simulink model "Cv_05_Problem_1"  (R2022b)
settings: Solver=VariableStepAuto  StartTime=0.0  StopTime=200  MaxStep=0.01  MinStep=0.001  RelTol=1e-3
libraries: slpidlib x5
settings Model: Creator=honza  LastModifiedBy=honza

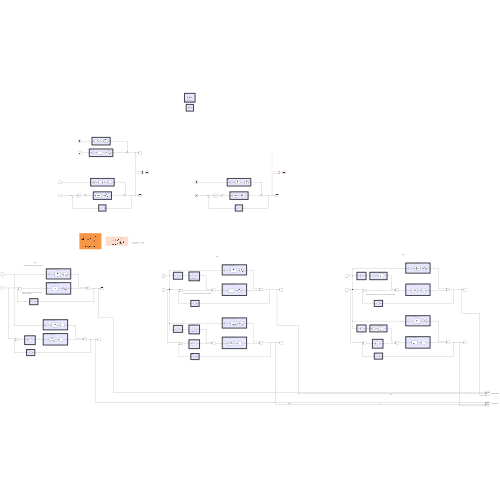
[thumbnail: Simulink's stored preview of the top-level diagram]
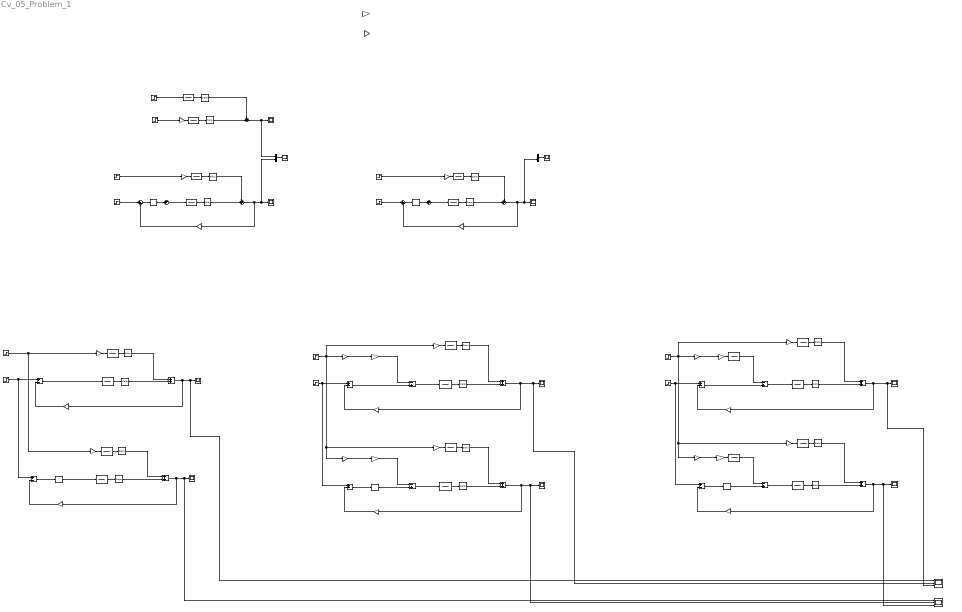
== system Cv_05_Problem_1 ==
  note: REGULOVANÁ
  note: NEREGULOVANÁ
  note: r0 = 0.35*15/(0.6*2)	= 4.375
      | Ti = 1.2*15			= 18
  note: Gt
  note: Gs
  note: Gd
  note: Gz
  note: Gs
  note: Gd
  note: Gf = -1/3
      |
      |
      |
      |
      | Gf = Gd/(Gt * Gs)
      | Ale jen to zesílení K
  note: Gs
  note: Gd
  note: Gz
  note: Gz = 1
  note: Gd = -(0.2 * e^-2s)/(10s + 1)
  note: Gt = 1
  note: Gz = 1
  note: Bod 2
  note: Bod 0
  note: Regulator vynechám, abych si ho mohl dopočítat a věděl co do něj zadat
  note: Bod 1
  note: Gd = -(0.2 * e^-2s)/(10s + 1)
  note: Gs = (0.6 * e^-2s)/(15s + 1)
  note: Gd = -(0.2 * e^-2s)/(10s + 1)
  note: Gr
  note: Gz = 1
  note: Gr
  note: Gt = 1
  note: Gf = -1/3
      |
      |
      |
      |
      | Gf = Gd/(Gt * Gs)
      | Ale jen to zesílení K
  note: Gz = 1
  note: Gz = 1
  note: Gs = (0.6 * e^-2s)/(15s + 1)
  note: Gs = (0.6 * e^-2s)/(15s + 1)
  note: Gd = -(0.2 * e^-2s)/(10s + 1)
  note: Gf = -1/3
      |
      |
      |
      |
      | Gf = Gd/(Gt * Gs)
      | Ale jen to zesílení K
  note: Gs = (0.6 * e^-2s)/(15s + 1)
  note: Regulator vynechám, abych si ho mohl dopočítat a věděl co do něj zadat
  note: Gs = (0.6 * e^-2s)/(15s + 1)
  note: Gz = 1
  note: Gd = -(0.2 * e^-2s)/(10s + 1)
  note: Gf = -1/3((15s + 1)/(10s + 1))
      |
      |
      |
      |
      | Gf = Gd/(Gt * Gs)
  note: Gf = -1/3((15s + 1)/(10s + 1))
  note: Gr
  note: Gd = -(0.2 * e^-2s)/(10s + 1)
  note: Gs = (0.6 * e^-2s)/(15s + 1)
  note: Gt = 1
  note: Gt = 1
  note: Otestujeme funkcnost bez kompenzace Gf (Gf = 0)
  note: Regulator vynechám, abych si ho mohl dopočítat a věděl co do něj zadat
  Add{,3,7,13} (4 alike) : Sum  Inputs=-+
  Add{1,4,6,9,11,14} (6 alike) : Sum
  Add{2,5,8,10,12,15} (6 alike) : Sum  Inputs=+-
  D3 : Step  Time=100  SampleTime=0
  D4 : Step  Time=100  SampleTime=0
  D5 : Step  Time=100  SampleTime=0
  Gain{,1,4,7..8,10,13,15..16,20..21,24,26} (13 alike) : Gain
  Gain{5,11,18..19,22} (5 alike) : Gain  Gain=-1/3
  Gain{2..3,6,9,12,14,17,23,25} (9 alike) : Gain  Gain=-1
  Mux : Mux  Inputs=2
  Mux1 : Mux  Inputs=2
  PID Controller{,1..4} (5 alike) : slpidlib/PID Controller  Controller=PI  Form=Ideal  TimeDomain=Continuous-time  UseExternalTs=off  SampleTime=-1  IntegratorMethod=Forward Euler  FilterMethod=Forward Euler  ControllerParametersSource=internal  P=4.375  I=1/18  UseKiTs=off  D=0  N=100  UseFilter=on  TunerSelectOption=Transfer Function Based (PID Tuner App)  InitialConditionSource=internal  InitialConditionForIntegrator=0  InitialConditionForFilter=0  DifferentiatorICPrevScaledInput=0  ExternalReset=none  TrackingMode=off  Kt=1  LimitOutput=off  SatLimitsSource=internal  UpperSaturationLimit=inf  LowerSaturationLimit=-inf  LinearizeAsGain=on  AntiWindupMode=none  Kb=1  LimitIntegrator=off  UpperIntegratorSaturationLimit=inf  LowerIntegratorSaturationLimit=-inf  POutMin=[]  POutMax=[]  IOutMin=[]  IOutMax=[]  DOutMin=[]  DOutMax=[]  NOutMin=[]  NOutMax=[]  SumOutMin=[]  SumOutMax=[]  SaturationOutMin=[]  SaturationOutMax=[]  PParamMin=[]  PParamMax=[]  IParamMin=[]  IParamMax=[]  DParamMin=[]  DParamMax=[]  NParamMin=[]  NParamMax=[]  KbParamMin=[]  KbParamMax=[]  KtParamMin=[]  KtParamMax=[]  KbOutMin=[]  KbOutMax=[]  KtOutMin=[]  KtOutMax=[]  IntegratorOutMin=[]  IntegratorOutMax=[]  FilterOutMin=[]  FilterOutMax=[]  SumI1OutMin=[]  SumI1OutMax=[]  SumI2OutMin=[]  SumI2OutMax=[]  SumI3OutMin=[]  SumI3OutMax=[]  SumI4OutMin=[]  SumI4OutMax=[]  SumDOutMin=[]  SumDOutMax=[]  DifferentiatorOutMin=[]  DifferentiatorOutMax=[]  FilterDiffOutCoefMin=[]  FilterDiffOutCoefMax=[]  ReciprocalOutMin=[]  ReciprocalOutMax=[]  SumDenOutMin=[]  SumDenOutMax=[]  SumNumOutMin=[]  SumNumOutMax=[]  DivideOutMin=[]  DivideOutMax=[]  UdiffTsProdOutMin=[]  UdiffTsProdOutMax=[]  NTsProdOutMin=[]  NTsProdOutMax=[]  UintegralTsProdOutMin=[]  UintegralTsProdOutMax=[]  UngainTsProdOutMin=[]  UngainTsProdOutMax=[]  ClampingZeroOutDataTypeStr=Inherit: Inherit via back propagation  ClampingZeroOutMin=[]  ClampingZeroOutMax=[]  FilterDenConstantOutDataTypeStr=Inherit: Inherit via back propagation  FilterDenConstantOutMin=[]  FilterDenConstantOutMax=[]  PCopyOutDataTypeStr=Inherit: Inherit via back propagation  PCopyOutMin=[]  PCopyOutMax=[]  NCopyOutDataTypeStr=Inherit: Inherit via back propagation  NCopyOutMin=[]  NCopyOutMax=[]  IntegratorContinuousStateAttributes=''  IntegratorStateMustResolveToSignalObject=off  IntegratorRTWStateStorageClass=Auto  FilterContinuousStateAttributes=''  FilterStateMustResolveToSignalObject=off  FilterRTWStateStorageClass=Auto  ParallelPVariant=Passthrough  IdealPVariant=InternalParameters  IVariant=InternalParameters  DVariant=Disabled  IntegratorVariant=Continuous  SatVariant=Disabled  AWVariant=Passthrough  PCopyVariant=Disabled  TRVariant=Disabled  FdbkBlocksVariant=Forward  IdealPFdbkVariant=Disabled  SatFdbkVariant=Disabled  DerivativeFilterVariant=Disabled  NVariant=Disabled  NCopyVariant=Disabled_SignalSpec  FilterICVariant=Disabled  IntegratorICVariant=InternalICs  ExternalResetVariant=Disabled  TRSumVariant=Passthrough  SumFdbkVariant=Disabled  SumVariant=Sum_PI  TsampFilterVariant=InternalTs  TsampNgainVariant=Passthrough  TsampIntegralVariant=Passthrough  ExternalSaturationOutDataTypeStr=Inherit: Same as second input
  Scope{,1..10} (11 alike) : Scope
  Scope11 : Scope  NumInputPorts=3
  Scope12 : Scope  NumInputPorts=3
  Step : Step  SampleTime=0
  Step1 : Step  Time=100  SampleTime=0
  Step2 : Step  Time=0  SampleTime=0
  Step3 : Step  Time=100  SampleTime=0
  Step4 : Step  SampleTime=0
  Step5 : Step  Time=100  SampleTime=0
  Sum : Sum  Inputs=|+-
  Sum1 : Sum  Inputs=++|
  Sum2 : Sum  Inputs=-+|
  Sum3 : Sum  Inputs=++|
  Sum4 : Sum  Inputs=|+-
  Sum5 : Sum  Inputs=++|
  Sum6 : Sum  Inputs=-+|
  Transfer Fcn{,2,4,6,8,10,14,16,18} (9 alike) : TransferFcn  Numerator=[0.6]  Denominator=[15 1]
  Transfer Fcn{1,3,5,7,9,11,15,17,19} (9 alike) : TransferFcn  Numerator=[0.2]  Denominator=[10 1]
  Transfer Fcn12 : TransferFcn  Numerator=[15 1]  Denominator=[10 1]
  Transfer Fcn13 : TransferFcn  Numerator=[15 1]  Denominator=[10 1]
  Transport Delay{,1..17} (18 alike) : TransportDelay  DelayTime=2
  W3 : Step  Time=0  SampleTime=0
  W4 : Step  Time=0  SampleTime=0
  W5 : Step  Time=0  SampleTime=0
  wires:
  Transfer Fcn/1 -> Transport Delay/1
  Transfer Fcn1/1 -> Transport Delay1/1
  Step/1 -> Sum/1
  Gain1/1 -> Sum/2
  Transport Delay/1 -> Sum1/2
  Sum1/1 -> Gain1/1, Mux/2, Scope/1
  Sum2/1 -> Transfer Fcn/1
  Sum/1 -> PID Controller/1
  Step2/1 -> Transfer Fcn2/1
  Transfer Fcn2/1 -> Transport Delay2/1
  Gain2/1 -> Transfer Fcn1/1
  Step1/1 -> Gain2/1
  Step3/1 -> Gain3/1
  Transfer Fcn3/1 -> Transport Delay3/1
  Gain3/1 -> Transfer Fcn3/1
  PID Controller/1 -> Sum2/2
  Transport Delay1/1 -> Sum1/1
  Transport Delay3/1 -> Sum3/2
  Transport Delay2/1 -> Sum3/1
  Sum3/1 -> Mux/1, Scope1/1
  Mux/1 -> Scope2/1
  Step5/1 -> Gain6/1
  Sum5/1 -> Gain4/1, Mux1/2, Scope3/1
  Sum4/1 -> PID Controller1/1
  Sum6/1 -> Transfer Fcn4/1
  Gain4/1 -> Sum4/2
  Step4/1 -> Sum4/1
  Transport Delay4/1 -> Sum5/2
  Transfer Fcn5/1 -> Transport Delay5/1
  Transport Delay5/1 -> Sum5/1
  Transfer Fcn4/1 -> Transport Delay4/1
  PID Controller1/1 -> Sum6/2
  Gain6/1 -> Transfer Fcn5/1
  Mux1/1 -> Scope4/1
  ? -> Mux1/1
  Add14/1 -> Scope12/3, Scope10/1, Gain16/1  "BOD 2"
  Add5/1 -> PID Controller3/1
  Add9/1 -> Scope12/2, Scope8/1, Gain10/1  "BOD 1"
  Transfer Fcn13/1 -> Add/1
  Gain17/1 -> Transfer Fcn11/1
  Gain14/1 -> Transfer Fcn19/1
  Gain7/1 -> Gain19/1
  Add11/1 -> Gain13/1, Scope12/1, Scope9/1  "BOD 0"
  Add12/1 -> Transfer Fcn18/1
  Gain22/1 -> Add3/1
  Add10/1 -> Add7/2
  Transfer Fcn12/1 -> Add13/1
  Gain24/1 -> Add8/2
  Gain13/1 -> Add12/2
  Add13/1 -> Transfer Fcn10/1
  Gain26/1 -> Gain11/1
  Gain15/1 -> Gain18/1
  Add15/1 -> Add13/2
  Gain21/1 -> Add5/2
  Transport Delay10/1 -> Add14/2
  Gain18/1 -> Transfer Fcn12/1
  Transfer Fcn17/1 -> Transport Delay15/1
  Transfer Fcn6/1 -> Transport Delay6/1
  Transport Delay14/1 -> Add9/2
  Add8/1 -> PID Controller2/1
  Transport Delay17/1 -> Add11/1
  Transfer Fcn19/1 -> Transport Delay17/1
  Gain10/1 -> Add10/2
  Transfer Fcn18/1 -> Transport Delay16/1
  Transport Delay15/1 -> Add9/1
  Add6/1 -> Gain24/1, Scope11/1, Scope7/1  "BOD 0"
  Transfer Fcn16/1 -> Transport Delay14/1
  Transport Delay11/1 -> Add14/1
  D3/1 -> Gain12/1, Gain20/1, Gain23/1, Gain26/1
  Transfer Fcn11/1 -> Transport Delay11/1
  Transport Delay8/1 -> Add4/2
  Transport Delay9/1 -> Add4/1
  W4/1 -> Add8/1, Add12/1
  Gain12/1 -> Transfer Fcn17/1
  Transport Delay13/1 -> Add6/1
  Add7/1 -> Transfer Fcn16/1
  Add4/1 -> Gain21/1, Scope11/2, Scope6/1  "BOD 1"
  Gain16/1 -> Add15/2
  Transport Delay7/1 -> Add1/1
  Gain11/1 -> Add7/1
  Transport Delay12/1 -> Add6/2
  Transport Delay16/1 -> Add11/2
  Gain23/1 -> Transfer Fcn9/1
  Add2/1 -> PID Controller4/1
  PID Controller4/1 -> Add/2
  Transfer Fcn8/1 -> Transport Delay8/1
  Transfer Fcn15/1 -> Transport Delay13/1
  W3/1 -> Add5/1, Add10/1
  PID Controller2/1 -> Transfer Fcn14/1
  Transfer Fcn10/1 -> Transport Delay10/1
  PID Controller3/1 -> Add3/2
  Gain25/1 -> Transfer Fcn15/1
  Add1/1 -> Scope11/3, Scope5/1, Gain8/1  "BOD 2"
  D4/1 -> Gain25/1, Gain14/1
  Gain19/1 -> Transfer Fcn13/1
  Transfer Fcn9/1 -> Transport Delay9/1
  Gain8/1 -> Add2/2
  Gain20/1 -> Gain22/1
  Add3/1 -> Transfer Fcn8/1
  D5/1 -> Gain7/1, Gain9/1, Gain17/1, Gain15/1
  W5/1 -> Add2/1, Add15/1
  Transport Delay6/1 -> Add1/2
  Add/1 -> Transfer Fcn6/1
  Transfer Fcn14/1 -> Transport Delay12/1
  Transfer Fcn7/1 -> Transport Delay7/1
  Gain9/1 -> Transfer Fcn7/1
